simulink model "P2_simulink_2"  (R2017a)
settings: Solver=VariableStepAuto  StartTime=0.0  StopTime=10.0  RelTol=1e-3
values from neighbouring files (symbols this model uses):
  b = 0.5    [P2_datos.m]
  L = 0.01    [P2_datos.m]
  M = 0.2    [P2_datos.m]
  R = 20    [P2_datos.m]
undefined symbols (not defined in the file or in its folder): i_eq, ki, ky, u_eq, y_eq
settings Model: Creator=joaqu  LastModifiedBy=feder

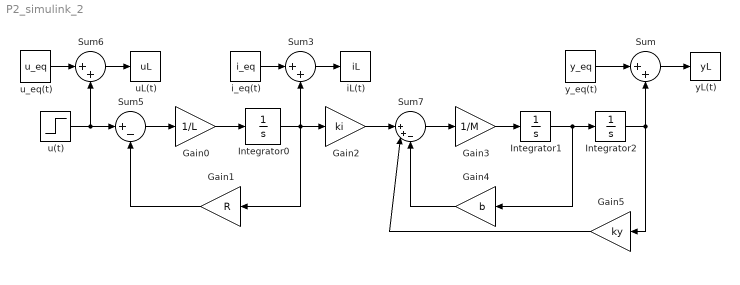
== system P2_simulink_2 ==
  Gain0 : Gain  Gain=1/L
  Gain1 : Gain  Gain=R
  Gain2 : Gain  Gain=ki
  Gain3 : Gain  Gain=1/M
  Gain4 : Gain  Gain=b
  Gain5 : Gain  Gain=ky
  Integrator0 : Integrator
  Integrator1 : Integrator
  Integrator2 : Integrator
  Sum : Sum  Inputs=|++
  Sum3 : Sum  Inputs=|++
  Sum5 : Sum  Inputs=|+-
  Sum6 : Sum  Inputs=|++
  Sum7 : Sum  Inputs=||++-
  iL(t) : ToWorkspace  VariableName=iL  SaveFormat=Timeseries  SampleTime=-1
  i_eq(t) : Constant  Value=i_eq
  u(t) : Step  Time=0  After=2  SampleTime=0
  uL(t) : ToWorkspace  VariableName=uL  SaveFormat=Timeseries  SampleTime=-1
  u_eq(t) : Constant  Value=u_eq
  yL(t) : ToWorkspace  VariableName=yL  SaveFormat=Timeseries  SampleTime=-1
  y_eq(t) : Constant  Value=y_eq
  wires:
  u_eq(t)/1 -> Sum6/1
  Sum6/1 -> uL(t)/1
  i_eq(t)/1 -> Sum3/1
  Sum3/1 -> iL(t)/1
  Sum/1 -> yL(t)/1
  Gain0/1 -> Integrator0/1
  u(t)/1 -> Sum6/2, Sum5/1
  Integrator0/1 -> Sum3/2, Gain2/1, Gain1/1
  Gain4/1 -> Sum7/3
  Integrator1/1 -> Integrator2/1, Gain4/1
  Gain3/1 -> Integrator1/1
  Sum5/1 -> Gain0/1
  Gain1/1 -> Sum5/2
  Integrator2/1 -> Sum/2, Gain5/1
  Sum7/1 -> Gain3/1
  Gain2/1 -> Sum7/1
  Gain5/1 -> Sum7/2
  y_eq(t)/1 -> Sum/1
